simulink model "task4"  (R2024a)
settings: Solver=VariableStepAuto  StartTime=0.0  StopTime=10.0  RelTol=1e-6
values from neighbouring files (symbols this model uses):
  A = [6, 0, -12, 6; 0, 6, -6, 12; -12, -6, 6, 0; 6, 12, 0, 6]    [main.m]
  B = [6; 12; 6; 4]    [main.m]
  C = [0, 0, 1, 0; 0, 0, 0, 1]    [main.m]
  CQi = inv([C; Q])    [main.m]
  D = [2; 2]    [main.m]
  G = [-3, 0; 0, -6]    [main.m]
  K = -acker(A, B, [-4, -1, -2, -3])    [main.m]
  Y = [1, 0; 1, 0]    [main.m]
undefined symbols (not defined in the file or in its folder): Q
settings Model: Creator=alexivanov  LastModifiedBy=alexivanov

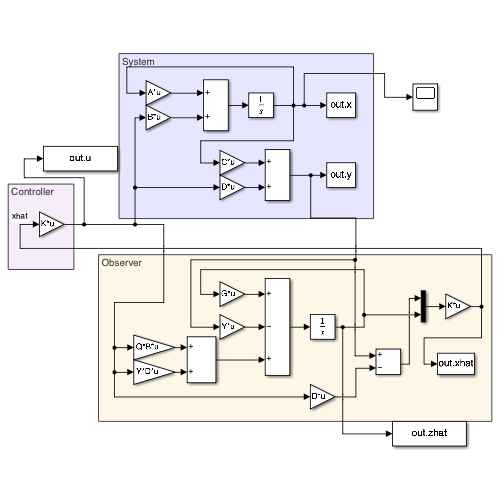
[thumbnail: Simulink's stored preview of the top-level diagram]
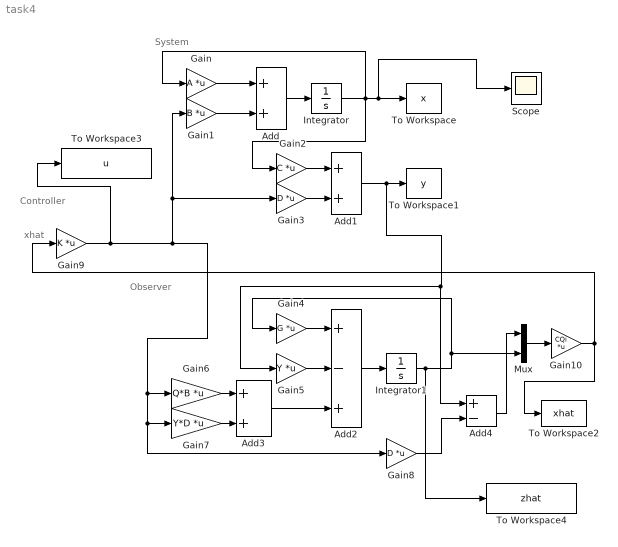
== system task4 ==
  note: Observer
  note: System
  note: xhat
  note: Controller
  Add : Sum
  Add1 : Sum
  Add2 : Sum  Inputs=+-+
  Add3 : Sum
  Add4 : Sum  Inputs=+-
  Gain : Gain  Gain=A  Multiplication=Matrix(K*u)
  Gain1 : Gain  Gain=B  Multiplication=Matrix(K*u)
  Gain10 : Gain  Gain=CQi  Multiplication=Matrix(K*u)
  Gain2 : Gain  Gain=C  Multiplication=Matrix(K*u)
  Gain3 : Gain  Gain=D  Multiplication=Matrix(K*u)
  Gain4 : Gain  Gain=G  Multiplication=Matrix(K*u)
  Gain5 : Gain  Gain=Y  Multiplication=Matrix(K*u)
  Gain6 : Gain  Gain=Q*B  Multiplication=Matrix(K*u)
  Gain7 : Gain  Gain=Y*D  Multiplication=Matrix(K*u)
  Gain8 : Gain  Gain=D  Multiplication=Matrix(K*u)
  Gain9 : Gain  Gain=K  Multiplication=Matrix(K*u)
  Integrator : Integrator  InitialCondition=[1, 1, 1, 1]
  Integrator1 : Integrator
  Mux : Mux  Inputs=2
  Scope : Scope
  To Workspace : ToWorkspace  VariableName=x  SampleTime=-1
  To Workspace1 : ToWorkspace  VariableName=y  SampleTime=-1
  To Workspace2 : ToWorkspace  VariableName=xhat  SampleTime=-1
  To Workspace3 : ToWorkspace  VariableName=u  SaveFormat=Timeseries  SampleTime=-1
  To Workspace4 : ToWorkspace  VariableName=zhat  SampleTime=-1
  wires:
  Gain2/1 -> Add1/1
  Gain3/1 -> Add1/2
  Gain1/1 -> Add/2
  Gain9/1 -> To Workspace3/1, Gain8/1, Gain7/1, Gain6/1, Gain3/1, Gain1/1
  Gain/1 -> Add/1
  Integrator/1 -> Gain2/1, Scope/1, To Workspace/1, Gain/1
  Add/1 -> Integrator/1
  Add1/1 -> Add4/1, Gain5/1, To Workspace1/1
  Add2/1 -> Integrator1/1
  Gain4/1 -> Add2/1
  Integrator1/1 -> To Workspace4/1, Gain4/1, Mux/2
  Gain5/1 -> Add2/2
  Gain6/1 -> Add3/1
  Gain7/1 -> Add3/2
  Add3/1 -> Add2/3
  Gain10/1 -> Gain9/1, To Workspace2/1
  Gain8/1 -> Add4/2
  Add4/1 -> Mux/1
  Mux/1 -> Gain10/1
